simulink model "lab1_ex2"  (R2025b)
settings: Solver=VariableStepAuto  StartTime=0.0  StopTime=10.0  RelTol=1e-3

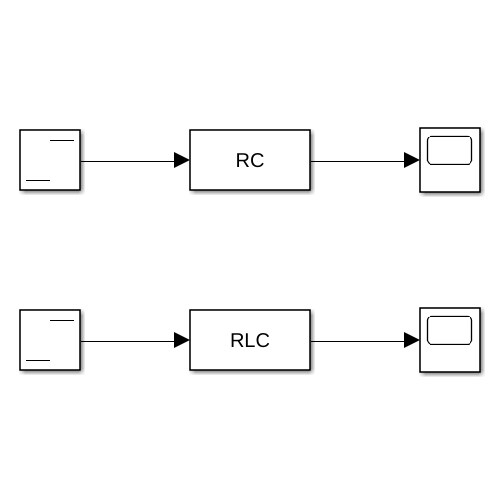
[thumbnail: Simulink's stored preview of the top-level diagram]
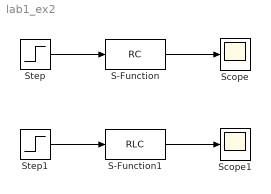
== system lab1_ex2 ==
  S-Function : S-Function  FunctionName=RC  Parameters=-1, 1, 1  SFunctionDeploymentMode=off  EnableBusSupport=off
  S-Function1 : S-Function  FunctionName=RLC  Parameters=[0,1e6;-1e3, -1e4];[0;1e3];[1, 0];  SFunctionDeploymentMode=off  EnableBusSupport=off
  Scope : Scope
      settings: ActiveDisplayYMinimum=-1  ActiveDisplayYMaximum=1
  Scope1 : Scope
      settings: ActiveDisplayYMinimum=-0.85724649574270639  ActiveDisplayYMaximum=3.11319787186706
  Step : Step  SampleTime=0
  Step1 : Step  SampleTime=0
  wires:
  Step/1 -> S-Function/1
  S-Function/1 -> Scope/1
  S-Function1/1 -> Scope1/1
  Step1/1 -> S-Function1/1
